simulink model "HW4_1b"  (R2023b)
settings: Solver=VariableStepAuto  StartTime=0.0  StopTime=100  RelTol=1e-3
model workspace (MAT data in the model file):
  a = Simulink.Parameter
  a.Value = 1
  a.DataType = 'auto'
  a.Complexity = 'real'
  a.Dimensions = [1 1]
  m = Simulink.Parameter
  m.Value = 20
  m.DataType = 'auto'
  m.Complexity = 'real'
  m.Dimensions = [1 1]
  theta_1_true = Simulink.Parameter
  theta_1_true.Value = 0.05
  theta_1_true.DataType = 'auto'
  theta_1_true.Complexity = 'real'
  theta_1_true.Dimensions = [1 1]
  theta_2_true = Simulink.Parameter
  theta_2_true.Value = 0.005
  theta_2_true.DataType = 'auto'
  theta_2_true.Complexity = 'real'
  theta_2_true.Dimensions = [1 1]
  theta_3_true = Simulink.Parameter
  theta_3_true.Value = 0.25
  theta_3_true.DataType = 'auto'
  theta_3_true.Complexity = 'real'
  theta_3_true.Dimensions = [1 1]
libraries: matrix_library x2
settings Model: Creator=kaleb  LastModifiedBy=kaleb

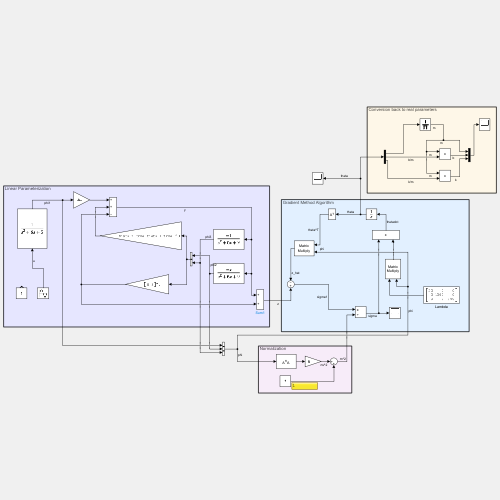
[thumbnail: Simulink's stored preview of the top-level diagram]
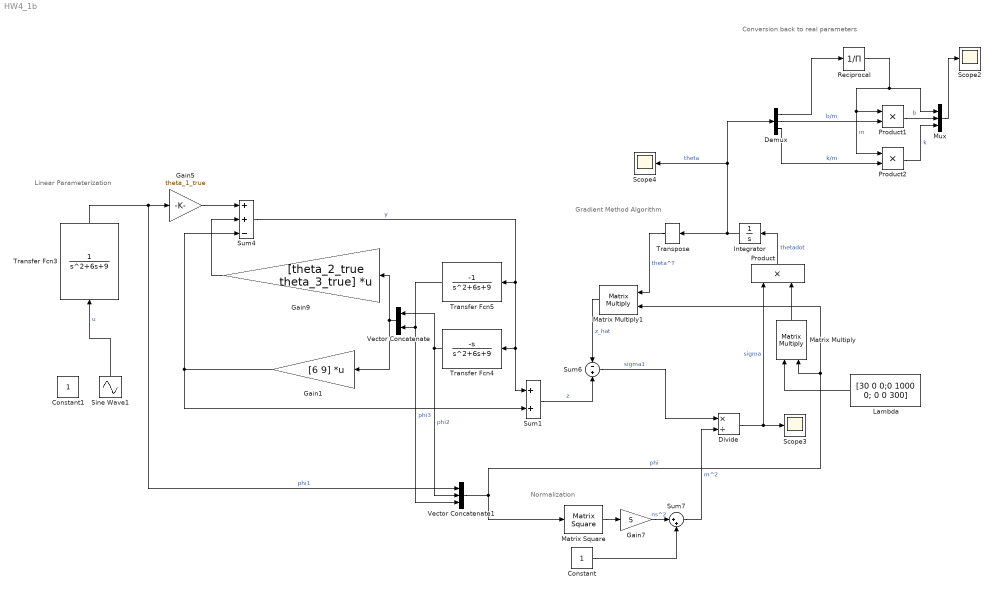
== system HW4_1b ==
  note: Gradient Method Algorithm
  note: Conversion back to real parameters
  note: Normalization
  note: Linear Parameterization
  Constant : Constant
  Constant1 : Constant
  Demux : Demux  Outputs=3
  Divide : Product  Inputs=*/
  Gain1 : Gain  Gain=[6 9]  Multiplication=Matrix(K*u)
  Gain5 : Gain  Gain=theta_1_true
  Gain7 : Gain  Gain=5
  Gain9 : Gain  Gain=[theta_2_true theta_3_true]  Multiplication=Matrix(K*u)
  Integrator : Integrator  InitialCondition=[0.1 0.1 0.3]
  Lambda : Constant  Value=[30 0 0;0 1000 0; 0 0 300]
  Matrix Square : matrix_library/Matrix Square  OutMin=[]  OutMax=[]
      settings: LibrarySourceBlock=|
      | simulink/Matrix
      | Operations/Matrix
      | Square
  Matrix Multiply : Product  Multiplication=Matrix(*)
  Matrix Multiply1 : Product  Multiplication=Matrix(*)
  Mux : Mux  Inputs=3
  Product : Product
  Product1 : Product
  Product2 : Product
  Reciprocal : Product  Inputs=/  OutMax=[10000]
  Scope2 : Scope
  Scope3 : Scope
  Scope4 : Scope
  Sine Wave1 : Sin  SampleTime=0
  Sum1 : Sum
  Sum4 : Sum  Inputs=++-
  Sum6 : Sum  Inputs=-+
  Sum7 : Sum  Inputs=|++
  Transfer Fcn3 : TransferFcn  Denominator=[1 6 9]
  Transfer Fcn4 : TransferFcn  Numerator=[-1 0]  Denominator=[1 6 9]
  Transfer Fcn5 : TransferFcn  Numerator=[-1]  Denominator=[1 6 9]
  Transpose : matrix_library/Transpose
  Vector Concatenate : Concatenate
  Vector Concatenate1 : Concatenate  NumInputs=3
  wires:
  Sine Wave1/1 -> Transfer Fcn3/1  "u"
  Transfer Fcn3/1 -> Vector Concatenate1/1, Gain5/1  "phi1"
  Sum4/1 -> Transfer Fcn5/1, Sum1/1, Transfer Fcn4/1  "y"
  Transfer Fcn4/1 -> Vector Concatenate/1, Vector Concatenate1/2  "phi2"
  Transfer Fcn5/1 -> Vector Concatenate/2, Vector Concatenate1/3  "phi3"
  Gain9/1 -> Sum4/2
  Vector Concatenate1/1 -> Matrix Multiply1/2, Matrix Multiply/2, Matrix Square/1  "phi"
  Matrix Multiply1/1 -> Sum6/1  "z_hat"
  Matrix Square/1 -> Gain7/1
  Constant/1 -> Sum7/2
  Sum7/1 -> Divide/2  "m^2"
  Gain7/1 -> Sum7/1  "ns^2"
  Sum6/1 -> Divide/1  "sigma1"
  Product/1 -> Integrator/1  "thetadot"
  Integrator/1 -> Transpose/1, Demux/1, Scope4/1  "theta"
  Transpose/1 -> Matrix Multiply1/1  "theta^T"
  Divide/1 -> Scope3/1, Product/1  "sigma"
  Demux/2 -> Product1/2  "b/m"
  Demux/3 -> Product2/2  "k/m"
  Reciprocal/1 -> Product1/1, Product2/1, Mux/1  "m"
  Product1/1 -> Mux/2  "b"
  Product2/1 -> Mux/3  "k"
  Mux/1 -> Scope2/1
  Matrix Multiply/1 -> Product/2
  Gain5/1 -> Sum4/1
  Demux/1 -> Reciprocal/1
  Vector Concatenate/1 -> Gain9/1, Gain1/1
  Gain1/1 -> Sum4/3, Sum1/2
  Sum1/1 -> Sum6/2  "z"
  Lambda/1 -> Matrix Multiply/1
